simulink model "Simulation_model"  (R2020a)
settings: Solver=VariableStepAuto  StartTime=0.0  StopTime=5  RelTol=1e-3
undefined symbols (not defined in the file): Acid, Lead
libraries: powerlib x33, simulink x4, powerlib_meascontrol x3, electricdrivelib x1, re_lib x1
settings Model: Creator=RazerGG  LastModifiedBy=venmo
settings SolverCC: AlgebraicLoopSolver=LineSearch

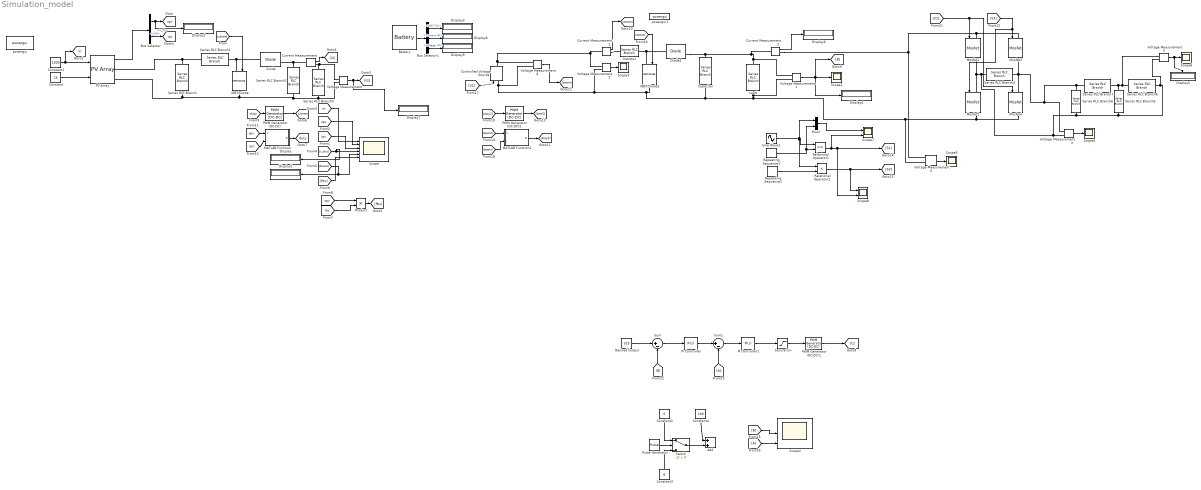
== system Simulation_model ==
  Add : Sum
  Battery : electricdrivelib/Extra Sources/Battery  BatType=Lead-Acid  ShowTempParam=off  ThermalPreset=no  ShowAgeParam=off  NomV=24  NomQ=50  SOC=0  Batt_Tr=30  PresetModel=on  MaxQ=52.0833  MinV=18  FullV=26.1316  Dis_rate=10  R=0.0048  Normal_OP=15.5139  expZone="[24.4342     0.166667]"  current=[6.5 13 32.5]  Units=Time  Tci=20  NomT=20  T2=-30  MaxQ2=4.8  FullV2=7.1  Normal_OP2=5.655  expZone2="[6.58           1]"  Rca=0.6  ti=2000  Dp=0  Neq0=0  Tsim=1e6  Ta1=25  Qeol=5.4*0.9  Reol=0.013333*1.2  Char_age=[2.3478, 3]  Dis_age=[2.3478, 10]  N1=1500  N2=10500  N3=1000  N4=1400  Ta2=45  N5=950
  Bus Selector : BusSelector  OutputSignals=V_PV,I_PV
  Bus Selector1 : BusSelector  OutputSignals=SOC (%),Current (A),Voltage (V)
  "Capacitor " : powerlib/Elements/Series RLC Branch  LConnTagsString=__new0  RConnTagsString=__new0  BranchType=C  Resistance=1  Inductance=1e-3  SetiL0=off  InitialCurrent=0  Capacitance=680e-6  Setx0=off  InitialVoltage=0  Measurements=None
  Constant : Constant  Value=25
  Constant1 : Constant  Value=1000
  Constant2 : Constant  Value=0
  Constant3 : Constant  Value=6
  Constant4 : Constant  Value=100
  Controlled Voltage Source : powerlib/Electrical Sources/Controlled Voltage Source  Initialize=on  Source_Type=AC  Amplitude=0  Phase=0  Frequency=0  Measurements=None
  Current Measurement : powerlib/Measurements/Current Measurement  PhasorSimulation=off  OutputType=Complex  PSBequivalent=0
  Current Measurement1 : powerlib/Measurements/Current Measurement  PhasorSimulation=off  OutputType=Complex  PSBequivalent=0
  Current Measurement2 : powerlib/Measurements/Current Measurement  PhasorSimulation=off  OutputType=Complex  PSBequivalent=0
  Desired Output : Constant  Value=325
  Diode : powerlib/Power Electronics/Diode  Ron=0.001  Lon=0  Vf=0.8  IC=0  UseSnubber=0  Rs=500  Cs=250e-9  Measurements=on
  Diode1 : powerlib/Power Electronics/Diode  Ron=0.001  Lon=0  Vf=0.8  IC=0  UseSnubber=off  Rs=500  Cs=250e-9  Measurements=on
  Display{,1..9} (10 alike) : Display
  IGBT/Diode : powerlib/Power Electronics/IGBT//Diode  Ron=1e-3  Rs=1e5  Cs=inf  Measurements=off
  IGBT/Diode1 : powerlib/Power Electronics/IGBT//Diode  Ron=1e-3  Rs=1e5  Cs=inf  Measurements=off
  "Inductor " : powerlib/Elements/Series RLC Branch  LConnTagsString=__new0  RConnTagsString=__new0  BranchType=L  Resistance=1  Inductance=150e-6  SetiL0=off  InitialCurrent=0  Capacitance=1e-6  Setx0=off  InitialVoltage=0  Measurements=None
  "Load " : powerlib/Elements/Series RLC Branch  LConnTagsString=__new0  RConnTagsString=__new0  BranchType=R  Resistance=100  Inductance=1e-3  SetiL0=off  InitialCurrent=0  Capacitance=1e-6  Setx0=off  InitialVoltage=0  Measurements=None
  MATLAB Function : MATLAB Function  TreatAsAtomicUnit=on
  MATLAB Function1 : MATLAB Function  TreatAsAtomicUnit=on
  Mosfet{1..4} (4 alike) : powerlib/Power Electronics/Mosfet  Ron=0.1  Lon=0  Rd=0.01  Vfd=0  IC=0  Rs=1e5  Cs=inf  Measurements=on
  Mux1 : Mux  Inputs=2
  PI Controller1 : simulink/Continuous/PID Controller  Controller=PI  Form=Parallel  TimeDomain=Continuous-time  UseExternalTs=off  SampleTime=-1  IntegratorMethod=Forward Euler  FilterMethod=Forward Euler  ControllerParametersSource=internal  P=0.4  I=80  D=0  UseFilter=on  N=100  TunerSelectOption=Transfer Function Based (PID Tuner App)  InitialConditionSource=internal  InitialConditionForIntegrator=0  InitialConditionForFilter=0  DifferentiatorICPrevScaledInput=0  ExternalReset=none  TrackingMode=off  Kt=1  LimitOutput=off  UpperSaturationLimit=inf  LowerSaturationLimit=-inf  LinearizeAsGain=on  AntiWindupMode=none  Kb=1  POutMin=[]  POutMax=[]  IOutMin=[]  IOutMax=[]  DOutMin=[]  DOutMax=[]  NOutMin=[]  NOutMax=[]  SumOutMin=[]  SumOutMax=[]  SaturationOutMin=[]  SaturationOutMax=[]  PParamMin=[]  PParamMax=[]  IParamMin=[]  IParamMax=[]  DParamMin=[]  DParamMax=[]  NParamMin=[]  NParamMax=[]  KbParamMin=[]  KbParamMax=[]  KtParamMin=[]  KtParamMax=[]  KbOutMin=[]  KbOutMax=[]  KtOutMin=[]  KtOutMax=[]  IntegratorOutMin=[]  IntegratorOutMax=[]  FilterOutMin=[]  FilterOutMax=[]  SumI1OutMin=[]  SumI1OutMax=[]  SumI2OutMin=[]  SumI2OutMax=[]  SumI3OutMin=[]  SumI3OutMax=[]  SumI4OutMin=[]  SumI4OutMax=[]  SumDOutMin=[]  SumDOutMax=[]  DifferentiatorOutMin=[]  DifferentiatorOutMax=[]  FilterDiffOutCoefMin=[]  FilterDiffOutCoefMax=[]  ReciprocalOutMin=[]  ReciprocalOutMax=[]  SumDenOutMin=[]  SumDenOutMax=[]  SumNumOutMin=[]  SumNumOutMax=[]  DivideOutMin=[]  DivideOutMax=[]  UdiffTsProdOutMin=[]  UdiffTsProdOutMax=[]  NTsProdOutMin=[]  NTsProdOutMax=[]  UintegralTsProdOutMin=[]  UintegralTsProdOutMax=[]  UngainTsProdOutMin=[]  UngainTsProdOutMax=[]  IntegratorContinuousStateAttributes=''  IntegratorStateMustResolveToSignalObject=off  IntegratorRTWStateStorageClass=Auto  FilterContinuousStateAttributes=''  FilterStateMustResolveToSignalObject=off  FilterRTWStateStorageClass=Auto  ParallelPVariant=InternalParameters  IdealPVariant=Disabled  IVariant=InternalParameters  DVariant=Disabled  IntegratorVariant=Continuous  SatVariant=Disabled  AWVariant=Passthrough  PCopyVariant=Disabled  TRVariant=Disabled  FdbkBlocksVariant=Forward  IdealPFdbkVariant=Disabled  SatFdbkVariant=Disabled  DerivativeFilterVariant=Disabled  NVariant=Disabled  NCopyVariant=Disabled_SignalSpec  FilterICVariant=Disabled  IntegratorICVariant=InternalICs  ExternalResetVariant=Disabled  TRSumVariant=Passthrough  SumFdbkVariant=Disabled  SumVariant=Sum_PI  TsampFilterVariant=InternalTs  TsampNgainVariant=Passthrough  TsampIntegralVariant=Passthrough
  PI Controller : simulink/Continuous/PID Controller  Controller=PI  Form=Parallel  TimeDomain=Continuous-time  UseExternalTs=off  SampleTime=-1  IntegratorMethod=Forward Euler  FilterMethod=Forward Euler  ControllerParametersSource=internal  P=0.4  I=80  D=0  UseFilter=on  N=100  TunerSelectOption=Transfer Function Based (PID Tuner App)  InitialConditionSource=internal  InitialConditionForIntegrator=0  InitialConditionForFilter=0  DifferentiatorICPrevScaledInput=0  ExternalReset=none  TrackingMode=off  Kt=1  LimitOutput=off  UpperSaturationLimit=inf  LowerSaturationLimit=-inf  LinearizeAsGain=on  AntiWindupMode=none  Kb=1  POutMin=[]  POutMax=[]  IOutMin=[]  IOutMax=[]  DOutMin=[]  DOutMax=[]  NOutMin=[]  NOutMax=[]  SumOutMin=[]  SumOutMax=[]  SaturationOutMin=[]  SaturationOutMax=[]  PParamMin=[]  PParamMax=[]  IParamMin=[]  IParamMax=[]  DParamMin=[]  DParamMax=[]  NParamMin=[]  NParamMax=[]  KbParamMin=[]  KbParamMax=[]  KtParamMin=[]  KtParamMax=[]  KbOutMin=[]  KbOutMax=[]  KtOutMin=[]  KtOutMax=[]  IntegratorOutMin=[]  IntegratorOutMax=[]  FilterOutMin=[]  FilterOutMax=[]  SumI1OutMin=[]  SumI1OutMax=[]  SumI2OutMin=[]  SumI2OutMax=[]  SumI3OutMin=[]  SumI3OutMax=[]  SumI4OutMin=[]  SumI4OutMax=[]  SumDOutMin=[]  SumDOutMax=[]  DifferentiatorOutMin=[]  DifferentiatorOutMax=[]  FilterDiffOutCoefMin=[]  FilterDiffOutCoefMax=[]  ReciprocalOutMin=[]  ReciprocalOutMax=[]  SumDenOutMin=[]  SumDenOutMax=[]  SumNumOutMin=[]  SumNumOutMax=[]  DivideOutMin=[]  DivideOutMax=[]  UdiffTsProdOutMin=[]  UdiffTsProdOutMax=[]  NTsProdOutMin=[]  NTsProdOutMax=[]  UintegralTsProdOutMin=[]  UintegralTsProdOutMax=[]  UngainTsProdOutMin=[]  UngainTsProdOutMax=[]  IntegratorContinuousStateAttributes=''  IntegratorStateMustResolveToSignalObject=off  IntegratorRTWStateStorageClass=Auto  FilterContinuousStateAttributes=''  FilterStateMustResolveToSignalObject=off  FilterRTWStateStorageClass=Auto  ParallelPVariant=InternalParameters  IdealPVariant=Disabled  IVariant=InternalParameters  DVariant=Disabled  IntegratorVariant=Continuous  SatVariant=Disabled  AWVariant=Passthrough  PCopyVariant=Disabled  TRVariant=Disabled  FdbkBlocksVariant=Forward  IdealPFdbkVariant=Disabled  SatFdbkVariant=Disabled  DerivativeFilterVariant=Disabled  NVariant=Disabled  NCopyVariant=Disabled_SignalSpec  FilterICVariant=Disabled  IntegratorICVariant=InternalICs  ExternalResetVariant=Disabled  TRSumVariant=Passthrough  SumFdbkVariant=Disabled  SumVariant=Sum_PI  TsampFilterVariant=InternalTs  TsampNgainVariant=Passthrough  TsampIntegralVariant=Passthrough
  PV Array : re_lib/Solar/PV Array  Npar=1  Nser=1  PlotType=array @ 1000 W/m2 & specified temperatures  S_vec="[ 1000  500  100 ]"  Temp_C_vec="[ 45 25  ]"  ModuleName=User-defined  PlotWhenSelected=off  Pm=30.072  Ncell=60  Voc=22.1  Isc=1.74  Vm=17.9  Im=1.68  beta_Voc_pc=-0.36099  alpha_Isc_pc=0.102  beta_Voc=-0.079779  alpha_Isc=0.0017748  IL=1.7715  I0=6.5275e-11  nI=0.59693  Rsh=1685.4807  Rs=0.8942  RobustModel=off  RobustCellTemperature=25  BAL=off  Tc=1e-6  Tfilter=5e-5
  PWM Generator (DC-DC) : powerlib_meascontrol/Pulse & Signal Generators/PWM Generator (DC-DC)  Fsw=5000  Ts=10e-6
  PWM Generator (DC-DC)1 : powerlib_meascontrol/Pulse & Signal Generators/PWM Generator (DC-DC)  Fsw=20e3  Ts=0
  PWM Generator (DC-DC)2 : powerlib_meascontrol/Pulse & Signal Generators/PWM Generator (DC-DC)  Fsw=5000  Ts=10e-6
  Product : Product
  Pulse Generator : DiscretePulseGenerator  PulseType=Time based  PulseWidth=50
  Relational Operator1 : RelationalOperator  OutDataTypeStr=boolean  RndMeth=Simplest
  Relational Operator2 : RelationalOperator  Operator=<  OutDataTypeStr=boolean  RndMeth=Simplest
  Repeating Sequence1 : simulink/Sources/Repeating Sequence  rep_seq_t=[0 0.5 1]/1000  rep_seq_y=[0 1 0]
  Repeating Sequence2 : simulink/Sources/Repeating Sequence  rep_seq_t=[0 0.5 1]/1000  rep_seq_y=[0 -1 0]
  Saturation : Saturate  UpperLimit=0.9  LowerLimit=0.1
  Scope : Scope  NumInputPorts=6
  Scope{1,3..6} (5 alike) : Scope
  Scope2 : Scope  NumInputPorts=3
  Scope7 : Scope  NumInputPorts=2
  Scope8 : Scope  NumInputPorts=2
  Series RLC Branch : powerlib/Elements/Series RLC Branch  LConnTagsString=__new0  RConnTagsString=__new0  BranchType=C  Resistance=1e-4  Inductance=1e-3  SetiL0=off  InitialCurrent=0  Capacitance=70e-6  Setx0=off  InitialVoltage=0  Measurements=None
  Series RLC Branch1 : powerlib/Elements/Series RLC Branch  LConnTagsString=__new0  RConnTagsString=__new0  BranchType=L  Resistance=0.1  Inductance=0.04e-3  SetiL0=off  InitialCurrent=0  Capacitance=100e-6  Setx0=off  InitialVoltage=0  Measurements=None
  Series RLC Branch2 : powerlib/Elements/Series RLC Branch  LConnTagsString=__new0  RConnTagsString=__new0  BranchType=C  Resistance=1e-4  Inductance=1e-3  SetiL0=off  InitialCurrent=0  Capacitance=470e-6  Setx0=off  InitialVoltage=0  Measurements=None
  Series RLC Branch3 : powerlib/Elements/Series RLC Branch  LConnTagsString=__new0  RConnTagsString=__new0  BranchType=R  Resistance=10  Inductance=1e-3  SetiL0=off  InitialCurrent=0  Capacitance=7e-4  Setx0=off  InitialVoltage=0  Measurements=None
  Series RLC Branch4 : powerlib/Elements/Series RLC Branch  LConnTagsString=__new0  RConnTagsString=__new0  BranchType=R  Resistance=50  Inductance=1e-3  SetiL0=off  InitialCurrent=0  Capacitance=1e-6  Setx0=off  InitialVoltage=0  Measurements=None
  Series RLC Branch5 : powerlib/Elements/Series RLC Branch  LConnTagsString=__new0  RConnTagsString=__new0  BranchType=C  Resistance=50  Inductance=10e-3  SetiL0=off  InitialCurrent=0  Capacitance=11e-6  Setx0=off  InitialVoltage=0  Measurements=None
  Series RLC Branch6 : powerlib/Elements/Series RLC Branch  LConnTagsString=__new0  RConnTagsString=__new0  BranchType=C  Resistance=50  Inductance=10e-3  SetiL0=off  InitialCurrent=0  Capacitance=11e-6  Setx0=off  InitialVoltage=0  Measurements=None
  Series RLC Branch7 : powerlib/Elements/Series RLC Branch  LConnTagsString=__new0  RConnTagsString=__new0  BranchType=L  Resistance=50  Inductance=2.8e-1  SetiL0=off  InitialCurrent=0  Capacitance=1e-6  Setx0=off  InitialVoltage=0  Measurements=None
  Series RLC Branch8 : powerlib/Elements/Series RLC Branch  LConnTagsString=__new0  RConnTagsString=__new0  BranchType=R  Resistance=100  Inductance=1e-3  SetiL0=off  InitialCurrent=0  Capacitance=1e-6  Setx0=off  InitialVoltage=0  Measurements=None
  Sine Wave1 : Sin  Frequency=2*pi*50  SampleTime=0
  Sum : Sum  Inputs=|+-
  Sum1 : Sum  Inputs=|+-
  Switch : Switch  Criteria=u2 > Threshold
  Voltage Measurement{,1..6} (7 alike) : powerlib/Measurements/Voltage Measurement  PhasorSimulation=off  OutputType=Complex  PSBequivalent=0
  powergui : powerlib/powergui  Priority=1  SimulationMode=Discrete  SampleTime=1e-5  frequency=60  Iterations=50  frequencyindice=0  Pbase=100e6  ErrMax=1e-4  UnitsV=kV  UnitsW=MW  buscounter=0  FunctionMessages=off  echomessages=off  EnableUseOfTLC=off  CurrentSourceSwitches=off  DisableSnubberDevices=off  DisableRonSwitches=off  DisableVfSwitches=off  DisplayEquations=off  AutomaticDiscreteSolvers=off  SolverType=Tustin/Backward Euler (TBE)  Interpol=off  ExternalGateDelay=off  methode=off  Ts=100  x0status=blocks  SPID=on  SwTol=0  HookPort=off  NonlinearTolerance=1e-4  nMaxIteration=100  ContinueOnMaxIteration=off  RestoreLinks=warning  ResistiveCurrentMeasurement=off  Frange=[0:2:500]  Ylog=off  Xlog=on  ShowGrid=off  save=off  variable=ZData  structure=OUTPUT_V  ZoomFFT=off  StartTime=0.0  cycles=1  DisplayStyle=1  fundamental=50  FreqAxis=off  MaxFrequency=1000  frequencyindicesteady=1  RmsSteady=1  display=off
  powergui1 : powerlib/powergui  Priority=1  SimulationMode=Continuous  SampleTime=50e-6  frequency=60  Iterations=50  frequencyindice=0  Pbase=100e6  ErrMax=1e-4  UnitsV=kV  UnitsW=MW  buscounter=0  FunctionMessages=off  echomessages=off  EnableUseOfTLC=off  CurrentSourceSwitches=off  DisableSnubberDevices=off  DisableRonSwitches=off  DisableVfSwitches=off  DisplayEquations=off  AutomaticDiscreteSolvers=off  SolverType=Tustin/Backward Euler (TBE)  Interpol=off  ExternalGateDelay=off  methode=off  Ts=10  x0status=blocks  SPID=off  SwTol=0  HookPort=off  NonlinearTolerance=1e-4  nMaxIteration=100  ContinueOnMaxIteration=off  RestoreLinks=warning  ResistiveCurrentMeasurement=off  Frange=[0:2:500]  Ylog=off  Xlog=on  ShowGrid=off  save=off  variable=ZData  structure=0  ZoomFFT=off  StartTime=0.0  cycles=1  DisplayStyle=1  fundamental=60  FreqAxis=off  MaxFrequency=1000  frequencyindicesteady=1  RmsSteady=1  display=off
  tag scope: duty=global, ipv=global, irr=global, s_boost=global, vpv=global
  wires:
  Constant/1 -> PV Array/2
  Constant1/1 -> [irr], PV Array/1
  PV Array/1 -> Bus Selector/1
  Bus Selector/1 -> Display2/1, [vpv]  "<V_PV>"
  Bus Selector/2 -> [ipv]  "<I_PV>"
  [s_boost] -> IGBT/Diode/1
  Voltage Measurement/1 -> Display7/1, [V2]
  Current Measurement/1 -> [I2]
  [irr] -> Scope/1
  [vpv] -> Scope/2
  [ipv] -> Scope/3
  [v_bus] -> Display/1, Scope/4
  [iboost] -> Display1/1, Scope/5
  [Ppv] -> Scope/6
  Product/1 -> [Ppv]
  [vpv] -> Product/1
  [ipv] -> Product/2
  PWM Generator (DC-DC)/1 -> [s_boost]
  [duty] -> PWM Generator (DC-DC)/1
  [vpv] -> MATLAB Function/1(V)
  [ipv] -> MATLAB Function/2(I)
  MATLAB Function/1(D) -> [duty]
  [S3] -> Mosfet2/1, Mosfet3/1
  Voltage Measurement2/1 -> Scope3/1
  Voltage Measurement5/1 -> Display5/1, Scope6/1
  PI Controller/1 -> Sum1/1
  Sum/1 -> PI Controller/1
  Voltage Measurement1/1 -> [B], Display4/1, Scope1/1
  Saturation/1 -> PWM Generator (DC-DC)1/1
  [A] -> Scope2/3
  Voltage Measurement3/1 -> Scope4/1
  [S1] -> Mosfet4/1, Mosfet1/1
  Constant3/1 -> Switch/3
  PWM Generator (DC-DC)1/1 -> [C]
  [A] -> Sum1/2
  Constant4/1 -> Add/1
  Voltage Measurement4/1 -> Scope5/1
  Sum1/1 -> PI Controller1/1
  [B] -> Sum/2
  [B] -> Scope2/2
  Desired Output/1 -> Sum/1
  Switch/1 -> Add/2
  Pulse Generator/1 -> Switch/2
  Constant2/1 -> Switch/1
  PI Controller1/1 -> Saturation/1
  Voltage Measurement6/1 -> [boostvt]
  [V2] -> Controlled Voltage Source/1
  Battery/1 -> Bus Selector1/1
  Bus Selector1/1 -> Display3/1  "<SOC (%)>"
  Bus Selector1/2 -> Display8/1  "<Current (A)>"
  Bus Selector1/3 -> Display9/1  "<Voltage (V)>"
  [boost2] -> IGBT/Diode1/1
  MATLAB Function1/1(D) -> [duty2]
  [boostit] -> MATLAB Function1/2(I)
  [boostvt] -> MATLAB Function1/1(V)
  Current Measurement1/1 -> [boostit]
  [duty2] -> PWM Generator (DC-DC)2/1
  PWM Generator (DC-DC)2/1 -> [boost2]
  Current Measurement2/1 -> Display6/1
  Mux1/1 -> Scope7/1
  Relational Operator2/1 -> Scope8/1, [S3]
  Relational Operator1/1 -> Scope8/2, [S1], Scope7/2
  Repeating Sequence1/1 -> Mux1/2, Relational Operator1/2
  Repeating Sequence2/1 -> Relational Operator2/2
  Sine Wave1/1 -> Relational Operator2/1, Relational Operator1/1, Mux1/1
  connections:
  Series RLC Branch/LConn1 -- Series RLC Branch1/RConn1 -- PV Array/RConn1
  IGBT/Diode/LConn1 -- Series RLC Branch1/LConn1 -- Diode/LConn1
  Series RLC Branch2/LConn1 -- Current Measurement/LConn1 -- Diode/RConn1
  Current Measurement/RConn1 -- Series RLC Branch3/LConn1 -- Voltage Measurement/LConn1
  Series RLC Branch7/RConn1 -- Series RLC Branch5/LConn1 -- Series RLC Branch8/LConn1 -- Voltage Measurement5/LConn1
  IGBT/Diode1/RConn1 -- Voltage Measurement6/LConn2 -- Controlled Voltage Source/LConn1 -- Voltage Measurement2/LConn2 -- Voltage Measurement1/LConn2 -- "Load "/RConn1 -- Voltage Measurement4/LConn2 -- Mosfet2/RConn1 -- Mosfet4/RConn1 -- "Capacitor "/RConn1
  Voltage Measurement3/LConn2 -- Series RLC Branch6/RConn1 -- Series RLC Branch5/RConn1 -- Voltage Measurement5/LConn2 -- Series RLC Branch8/RConn1 -- Mosfet1/RConn1 -- Mosfet2/LConn1 -- Series RLC Branch4/LConn1
  Mosfet4/LConn1 -- Mosfet3/RConn1 -- Series RLC Branch6/LConn1 -- Series RLC Branch7/LConn1 -- Voltage Measurement3/LConn1 -- Series RLC Branch4/RConn1
  "Load "/LConn1 -- Voltage Measurement1/LConn1 -- Current Measurement2/LConn1 -- Diode1/RConn1 -- "Capacitor "/LConn1
  "Inductor "/RConn1 -- IGBT/Diode1/LConn1 -- Diode1/LConn1
  "Inductor "/LConn1 -- Current Measurement1/RConn1
  Series RLC Branch2/RConn1 -- Series RLC Branch/RConn1 -- PV Array/RConn2 -- IGBT/Diode/RConn1 -- Voltage Measurement/LConn2 -- Series RLC Branch3/RConn1
  Current Measurement1/LConn1 -- Voltage Measurement6/LConn1 -- Controlled Voltage Source/RConn1 -- Voltage Measurement2/LConn1
  Voltage Measurement4/LConn1 -- Current Measurement2/RConn1 -- Mosfet3/LConn1 -- Mosfet1/LConn1

== matlab function Simulation_model/MATLAB Function ==
  data: V input; D output; I input
function D = DutyRatio(V,I)

Dmax = 0.6;
Dmin = 0;
Dinit = 0.6;
deltaD = 125e-6;
persistent Vold Pold Dold

if isempty(Vold)
    Vold = 20;
    Pold = 100;
    Dold = Dinit;
end

P = V*I;
dV = V-Vold;
dP = P-Pold;

if dP ~= 0
    if dP<0
        if dV<0
            D = Dold - deltaD;
        else
            D = Dold + deltaD;
        end
    else
        if dV<0
            D = Dold + deltaD;
        else
            D = Dold - deltaD;
        end
    end
else D = Dold;
end

if D >= Dmax || D <= Dmin
    D = Dold;
end

Dold = D;
Vold = V;
Pold = P;

== matlab function Simulation_model/MATLAB Function1 ==
  data: V input; D output; I input
function D = DutyRatio(V,I)

Dmax = 0.95;
Dmin = 0;
Dinit = 0.95;
deltaD = 125e-6;
persistent Vold Pold Dold

if isempty(Vold)
    Vold = 20;
    Pold = 100;
    Dold = Dinit;
end

P = V*I;
dV = V-Vold;
dP = P-Pold;

if dP ~= 0
    if dP<0
        if dV<0
            D = Dold - deltaD;
        else
            D = Dold + deltaD;
        end
    else
        if dV<0
            D = Dold + deltaD;
        else
            D = Dold - deltaD;
        end
    end
else D = Dold;
end

if D >= Dmax || D <= Dmin
    D = Dold;
end

Dold = D;
Vold = V;
Pold = P;
